simulink model "PONG"  (R2018b)
settings: Solver=VariableStepAuto  StartTime=0.0  StopTime=10  RelTol=1e-3
libraries: simulink_extras x28
(part 3 of 3)

== system PONG/Paddle DEMUXER1/1PaddleDEMUXER2 ==
  PA : Inport
  PB : Inport  Port=2
  PC : Inport  Port=3
  Logical Operator{,1..7} (8 alike) : Logic  Inputs=3  IconShape=distinctive  AllPortsSameDT=off  OutDataTypeStr=boolean
  NOT : Logic  Operator=NOT  IconShape=distinctive  AllPortsSameDT=off  OutDataTypeStr=boolean
  NOT1 : Logic  Operator=NOT  IconShape=distinctive  AllPortsSameDT=off  OutDataTypeStr=boolean
  NOT2 : Logic  Operator=NOT  IconShape=distinctive  AllPortsSameDT=off  OutDataTypeStr=boolean
  Out1 : Outport
  Out2 : Outport  Port=2
  Out3 : Outport  Port=3
  Out4 : Outport  Port=4
  Out5 : Outport  Port=5
  Out6 : Outport  Port=6
  Out7 : Outport  Port=7
  Out8 : Outport  Port=8
  wires:
  PB/1 -> NOT1/1, Logical Operator3/2, Logical Operator7/2, Logical Operator6/2, Logical Operator2/2
  PC/1 -> NOT/1, Logical Operator1/3, Logical Operator3/3, Logical Operator5/3, Logical Operator7/1
  NOT2/1 -> Logical Operator1/1, Logical Operator2/1, Logical Operator3/1, Logical Operator/1
  NOT1/1 -> Logical Operator/2, Logical Operator1/2, Logical Operator4/2, Logical Operator5/2
  NOT/1 -> Logical Operator4/3, Logical Operator6/3, Logical Operator2/3, Logical Operator/3
  PA/1 -> NOT2/1, Logical Operator4/1, Logical Operator5/1, Logical Operator7/3, Logical Operator6/1
  Logical Operator4/1 -> Out5/1
  Logical Operator5/1 -> Out6/1
  Logical Operator6/1 -> Out7/1
  Logical Operator7/1 -> Out8/1
  Logical Operator2/1 -> Out3/1
  Logical Operator3/1 -> Out4/1
  Logical Operator1/1 -> Out2/1
  Logical Operator/1 -> Out1/1

== system PONG/Paddle0/Atomic Subsystem ==
  Ctrl : Inport
  CLK : Inport  Port=2
  Constant : Constant  OutDataTypeStr=boolean
  J-K Flip-Flop : simulink_extras/Flip Flops/J-K Flip-Flop  initial_condition=0
      settings: SourceProductName=Simulink
  J-K Flip-Flop1 : simulink_extras/Flip Flops/J-K Flip-Flop  initial_condition=0
      settings: SourceProductName=Simulink
  J-K Flip-Flop2 : simulink_extras/Flip Flops/J-K Flip-Flop  initial_condition=0
      settings: SourceProductName=Simulink
  Logical Operator : Logic  Operator=XOR  IconShape=distinctive  AllPortsSameDT=off  OutDataTypeStr=boolean
  Logical Operator1 : Logic  Operator=XOR  IconShape=distinctive  AllPortsSameDT=off  OutDataTypeStr=boolean
  Scope : Scope  NumInputPorts=3
  PA0 : Outport
  PB0 : Outport  Port=2
  PC0 : Outport  Port=3
  wires:
  CLK/1 -> J-K Flip-Flop/2
  J-K Flip-Flop/1 -> Logical Operator/1, Scope/1, PC0/1
  J-K Flip-Flop2/1 -> Scope/3, PA0/1
  J-K Flip-Flop1/1 -> Logical Operator1/1, Scope/2, PB0/1
  Ctrl/1 -> Logical Operator1/2, Logical Operator/2
  Logical Operator/1 -> J-K Flip-Flop1/2
  Logical Operator1/1 -> J-K Flip-Flop2/2
  Constant/1 -> J-K Flip-Flop2/3, J-K Flip-Flop2/1, J-K Flip-Flop1/3, J-K Flip-Flop1/1, J-K Flip-Flop/3, J-K Flip-Flop/1

== system PONG/Paddle0/Atomic Subsystem1 ==
  PA0 : Inport
  PB0 : Inport  Port=2
  PC0 : Inport  Port=3
  Logical Operator1 : Logic  Operator=XOR  IconShape=distinctive  AllPortsSameDT=off  OutDataTypeStr=boolean
  Logical Operator2 : Logic  Operator=NOT  IconShape=distinctive  AllPortsSameDT=off  OutDataTypeStr=boolean
  Logical Operator3 : Logic  Operator=XOR  IconShape=distinctive  AllPortsSameDT=off  OutDataTypeStr=boolean
  Logical Operator4 : Logic  IconShape=distinctive  AllPortsSameDT=off  OutDataTypeStr=boolean
  Scope : Scope  NumInputPorts=3
  PA1 : Outport
  PB1 : Outport  Port=2
  PC1 : Outport  Port=3
  wires:
  Logical Operator2/1 -> Scope/3, PC1/1
  PB0/1 -> Logical Operator4/1, Logical Operator1/1
  PA0/1 -> Logical Operator3/1
  Logical Operator3/1 -> Scope/1, PA1/1
  Logical Operator1/1 -> Scope/2, PB1/1
  Logical Operator4/1 -> Logical Operator3/2
  PC0/1 -> Logical Operator4/2, Logical Operator1/2, Logical Operator2/1

== system PONG/Paddle0/Atomic Subsystem2 ==
  PA0 : Inport
  PB0 : Inport  Port=2
  PC0 : Inport  Port=3
  Logical Operator1 : Logic  Operator=NXOR  IconShape=distinctive  AllPortsSameDT=off  OutDataTypeStr=boolean
  Logical Operator2 : Logic  Operator=NOT  IconShape=distinctive  AllPortsSameDT=off  OutDataTypeStr=boolean
  Logical Operator3 : Logic  Operator=NXOR  IconShape=distinctive  AllPortsSameDT=off  OutDataTypeStr=boolean
  Logical Operator4 : Logic  Operator=OR  IconShape=distinctive  AllPortsSameDT=off  OutDataTypeStr=boolean
  Scope : Scope  NumInputPorts=3
  PA1 : Outport
  PB1 : Outport  Port=2
  PC1 : Outport  Port=3
  wires:
  PC0/1 -> Logical Operator2/1, Logical Operator1/2, Logical Operator4/2
  Logical Operator4/1 -> Logical Operator3/2
  Logical Operator1/1 -> PB1/1, Scope/2
  Logical Operator3/1 -> PA1/1, Scope/1
  PA0/1 -> Logical Operator3/1
  PB0/1 -> Logical Operator1/1, Logical Operator4/1
  Logical Operator2/1 -> PC1/1, Scope/3

== system PONG/Paddle0/Atomic Subsystem3 ==
  CLK : Inport
  Ctrl : Inport  Port=2
  Constant : Constant  OutDataTypeStr=boolean
  J-K Flip-Flop : simulink_extras/Flip Flops/J-K Flip-Flop  initial_condition=0
      settings: SourceProductName=Simulink
  J-K Flip-Flop1 : simulink_extras/Flip Flops/J-K Flip-Flop  initial_condition=0
      settings: SourceProductName=Simulink
  J-K Flip-Flop2 : simulink_extras/Flip Flops/J-K Flip-Flop  initial_condition=1
      settings: SourceProductName=Simulink
  Logical Operator12 : Logic  Operator=OR  IconShape=distinctive  AllPortsSameDT=off  OutDataTypeStr=boolean
  Logical Operator13 : Logic  Operator=OR  IconShape=distinctive  AllPortsSameDT=off  OutDataTypeStr=boolean
  Logical Operator{8..9,14..15} (4 alike) : Logic  IconShape=distinctive  AllPortsSameDT=off  OutDataTypeStr=boolean
  NOT1 : Logic  Operator=NOT  IconShape=distinctive  AllPortsSameDT=off  OutDataTypeStr=boolean
  Scope : Scope  NumInputPorts=3
  PA0 : Outport
  PB0 : Outport  Port=2
  PC0 : Outport  Port=3
  wires:
  J-K Flip-Flop1/2 -> Logical Operator15/1
  Logical Operator12/1 -> J-K Flip-Flop1/3, J-K Flip-Flop1/1
  Logical Operator8/1 -> Logical Operator12/1, Logical Operator14/1
  J-K Flip-Flop2/1 -> PA0/1, Scope/3
  J-K Flip-Flop1/1 -> Scope/2, PB0/1, Logical Operator14/2
  NOT1/1 -> Logical Operator9/2
  Logical Operator13/1 -> J-K Flip-Flop2/1, J-K Flip-Flop2/3
  Logical Operator9/1 -> Logical Operator15/2, Logical Operator12/2
  Logical Operator14/1 -> Logical Operator13/1
  Constant/1 -> J-K Flip-Flop/1, J-K Flip-Flop/3
  CLK/1 -> J-K Flip-Flop2/2, J-K Flip-Flop1/2, J-K Flip-Flop/2
  Ctrl/1 -> Logical Operator8/1, NOT1/1
  J-K Flip-Flop/1 -> Scope/1, PC0/1, Logical Operator8/2
  Logical Operator15/1 -> Logical Operator13/2
  J-K Flip-Flop/2 -> Logical Operator9/1

== system PONG/Paddle1/Atomic Subsystem1 ==
  PA0 : Inport
  PB0 : Inport  Port=2
  PC0 : Inport  Port=3
  Logical Operator1 : Logic  Operator=XOR  IconShape=distinctive  AllPortsSameDT=off  OutDataTypeStr=boolean
  Logical Operator2 : Logic  Operator=NOT  IconShape=distinctive  AllPortsSameDT=off  OutDataTypeStr=boolean
  Logical Operator3 : Logic  Operator=XOR  IconShape=distinctive  AllPortsSameDT=off  OutDataTypeStr=boolean
  Logical Operator4 : Logic  IconShape=distinctive  AllPortsSameDT=off  OutDataTypeStr=boolean
  Scope : Scope  NumInputPorts=3
  PA1 : Outport
  PB1 : Outport  Port=2
  PC1 : Outport  Port=3
  wires:
  PC0/1 -> Logical Operator2/1, Logical Operator1/2, Logical Operator4/2
  Logical Operator4/1 -> Logical Operator3/2
  Logical Operator1/1 -> PB1/1, Scope/2
  Logical Operator3/1 -> PA1/1, Scope/1
  PA0/1 -> Logical Operator3/1
  PB0/1 -> Logical Operator1/1, Logical Operator4/1
  Logical Operator2/1 -> PC1/1, Scope/3

== system PONG/Paddle1/Atomic Subsystem2 ==
  PA0 : Inport
  PB0 : Inport  Port=2
  PC0 : Inport  Port=3
  Logical Operator1 : Logic  Operator=NXOR  IconShape=distinctive  AllPortsSameDT=off  OutDataTypeStr=boolean
  Logical Operator2 : Logic  Operator=NOT  IconShape=distinctive  AllPortsSameDT=off  OutDataTypeStr=boolean
  Logical Operator3 : Logic  Operator=NXOR  IconShape=distinctive  AllPortsSameDT=off  OutDataTypeStr=boolean
  Logical Operator4 : Logic  Operator=OR  IconShape=distinctive  AllPortsSameDT=off  OutDataTypeStr=boolean
  Scope : Scope  NumInputPorts=3
  PA1 : Outport
  PB1 : Outport  Port=2
  PC1 : Outport  Port=3
  wires:
  Logical Operator2/1 -> Scope/3, PC1/1
  PB0/1 -> Logical Operator4/1, Logical Operator1/1
  PA0/1 -> Logical Operator3/1
  Logical Operator3/1 -> Scope/1, PA1/1
  Logical Operator1/1 -> Scope/2, PB1/1
  Logical Operator4/1 -> Logical Operator3/2
  PC0/1 -> Logical Operator4/2, Logical Operator1/2, Logical Operator2/1

== system PONG/Paddle1/Atomic Subsystem3 ==
  CLK : Inport
  Ctrl : Inport  Port=2
  Constant : Constant  OutDataTypeStr=boolean
  J-K Flip-Flop : simulink_extras/Flip Flops/J-K Flip-Flop  initial_condition=1
      settings: SourceProductName=Simulink
  J-K Flip-Flop1 : simulink_extras/Flip Flops/J-K Flip-Flop  initial_condition=1
      settings: SourceProductName=Simulink
  J-K Flip-Flop2 : simulink_extras/Flip Flops/J-K Flip-Flop  initial_condition=0
      settings: SourceProductName=Simulink
  Logical Operator12 : Logic  Operator=OR  IconShape=distinctive  AllPortsSameDT=off  OutDataTypeStr=boolean
  Logical Operator13 : Logic  Operator=OR  IconShape=distinctive  AllPortsSameDT=off  OutDataTypeStr=boolean
  Logical Operator{8..9,14..15} (4 alike) : Logic  IconShape=distinctive  AllPortsSameDT=off  OutDataTypeStr=boolean
  NOT1 : Logic  Operator=NOT  IconShape=distinctive  AllPortsSameDT=off  OutDataTypeStr=boolean
  Scope : Scope  NumInputPorts=3
  PA0 : Outport
  PB0 : Outport  Port=2
  PC0 : Outport  Port=3
  wires:
  J-K Flip-Flop/2 -> Logical Operator9/1
  Logical Operator15/1 -> Logical Operator13/2
  J-K Flip-Flop/1 -> Logical Operator8/2, PC0/1, Scope/1
  Ctrl/1 -> NOT1/1, Logical Operator8/1
  CLK/1 -> J-K Flip-Flop/2, J-K Flip-Flop1/2, J-K Flip-Flop2/2
  Constant/1 -> J-K Flip-Flop/3, J-K Flip-Flop/1
  Logical Operator14/1 -> Logical Operator13/1
  Logical Operator9/1 -> Logical Operator15/2, Logical Operator12/2
  Logical Operator13/1 -> J-K Flip-Flop2/3, J-K Flip-Flop2/1
  NOT1/1 -> Logical Operator9/2
  J-K Flip-Flop1/1 -> Logical Operator14/2, PB0/1, Scope/2
  J-K Flip-Flop2/1 -> Scope/3, PA0/1
  Logical Operator8/1 -> Logical Operator14/1, Logical Operator12/1
  Logical Operator12/1 -> J-K Flip-Flop1/1, J-K Flip-Flop1/3
  J-K Flip-Flop1/2 -> Logical Operator15/1

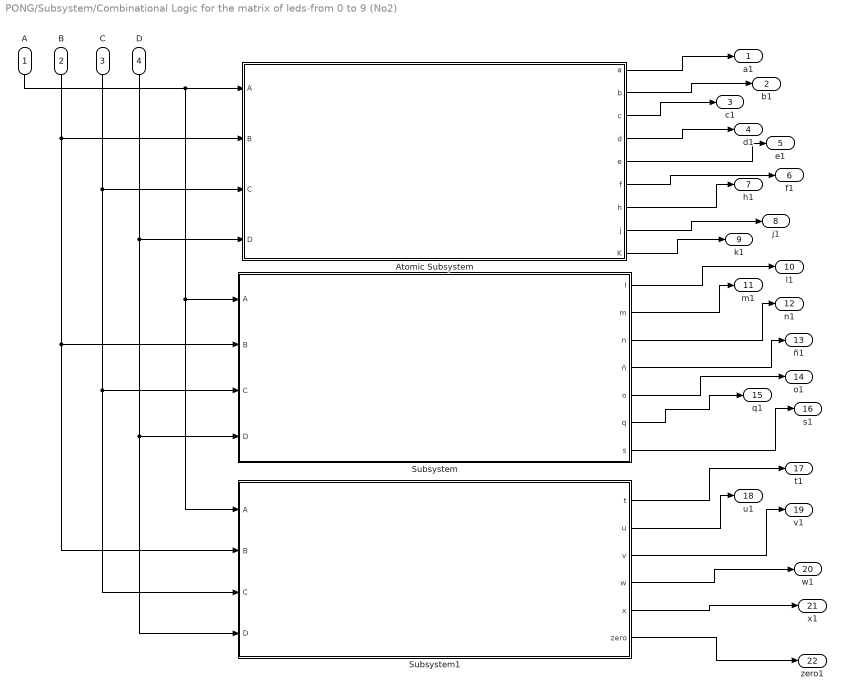
== system PONG/Subsystem/Combinational Logic for the matrix of leds-from 0 to 9 (No2) ==
  A : Inport
  B : Inport  Port=2
  C : Inport  Port=3
  D : Inport  Port=4
  Atomic Subsystem : Subsystem  TreatAsAtomicUnit=on
  Subsystem : Subsystem
  Subsystem1 : Subsystem
  a1 : Outport
  b1 : Outport  Port=2
  c1 : Outport  Port=3
  d1 : Outport  Port=4
  e1 : Outport  Port=5
  f1 : Outport  Port=6
  h1 : Outport  Port=7
  j1 : Outport  Port=8
  k1 : Outport  Port=9
  l1 : Outport  Port=10
  m1 : Outport  Port=11
  n1 : Outport  Port=12
  ñ1 : Outport  Port=13
  o1 : Outport  Port=14
  q1 : Outport  Port=15
  s1 : Outport  Port=16
  t1 : Outport  Port=17
  u1 : Outport  Port=18
  v1 : Outport  Port=19
  w1 : Outport  Port=20
  x1 : Outport  Port=21
  zero1 : Outport  Port=22
  wires:
  Atomic Subsystem/1(a) -> a1/1
  Atomic Subsystem/2(b) -> b1/1
  Atomic Subsystem/3(c) -> c1/1
  Atomic Subsystem/4(d) -> d1/1
  Atomic Subsystem/5(e) -> e1/1
  Atomic Subsystem/6(f) -> f1/1
  Atomic Subsystem/7(h) -> h1/1
  Atomic Subsystem/8(j) -> j1/1
  Atomic Subsystem/9(K) -> k1/1
  Subsystem/1(l) -> l1/1
  Subsystem/2(m) -> m1/1
  Subsystem/3(n) -> n1/1
  Subsystem/4(ñ) -> ñ1/1
  Subsystem/5(o) -> o1/1
  Subsystem/6(q) -> q1/1
  Subsystem/7(s) -> s1/1
  Subsystem1/1(t) -> t1/1
  Subsystem1/2(u) -> u1/1
  Subsystem1/3(v) -> v1/1
  Subsystem1/4(w) -> w1/1
  Subsystem1/5(x) -> x1/1
  A/1 -> Subsystem1/1(A), Subsystem/1(A), Atomic Subsystem/1(A)
  B/1 -> Subsystem1/2(B), Subsystem/2(B), Atomic Subsystem/2(B)
  C/1 -> Subsystem1/3(C), Subsystem/3(C), Atomic Subsystem/3(C)
  D/1 -> Subsystem1/4(D), Subsystem/4(D), Atomic Subsystem/4(D)
  Subsystem1/6(zero) -> zero1/1

== system PONG/Subsystem/Counter from 0 to 9 ==
  EN : Inport
  CLK : Inport  Port=2
  " B JK FLIP FLOP" : simulink_extras/Flip Flops/J-K Flip-Flop  initial_condition=0
      settings: SourceProductName=Simulink
  A JK FLIP FLOP : simulink_extras/Flip Flops/J-K Flip-Flop  initial_condition=0
      settings: SourceProductName=Simulink
  C Jk flip flop : simulink_extras/Flip Flops/J-K Flip-Flop  initial_condition=0
      settings: SourceProductName=Simulink
  D jk flip-flop : simulink_extras/Flip Flops/J-K Flip-Flop  initial_condition=0
      settings: SourceProductName=Simulink
  Display3 : Display
      settings: Format=binary (Stored Integer)
  Logical Operator : Logic  IconShape=distinctive  AllPortsSameDT=off  OutDataTypeStr=boolean
  Logical Operator1 : Logic  IconShape=distinctive  AllPortsSameDT=off  OutDataTypeStr=boolean
  Logical Operator2 : Logic  Inputs=3  IconShape=distinctive  AllPortsSameDT=off  OutDataTypeStr=boolean
  Mux : Mux
  A : Outport
  B : Outport  Port=2
  C : Outport  Port=3
  D : Outport  Port=4
  wires:
  C Jk flip flop/1 -> Logical Operator2/2, Logical Operator1/2, C/1, Mux/3
  Mux/1 -> Display3/1
  Logical Operator2/1 -> A JK FLIP FLOP/1
  A JK FLIP FLOP/1 -> A/1, Mux/1
  Logical Operator1/1 -> " B JK FLIP FLOP"/3, " B JK FLIP FLOP"/1
  Logical Operator/1 -> C Jk flip flop/1
  " B JK FLIP FLOP"/1 -> Logical Operator2/3, B/1, Mux/2
  CLK/1 -> A JK FLIP FLOP/2, " B JK FLIP FLOP"/2, C Jk flip flop/2, D jk flip-flop/2
  D jk flip-flop/1 -> Logical Operator2/1, A JK FLIP FLOP/3, Logical Operator1/1, Logical Operator/1, D/1, Mux/4, C Jk flip flop/3
  EN/1 -> D jk flip-flop/3, D jk flip-flop/1
  A JK FLIP FLOP/2 -> Logical Operator/2

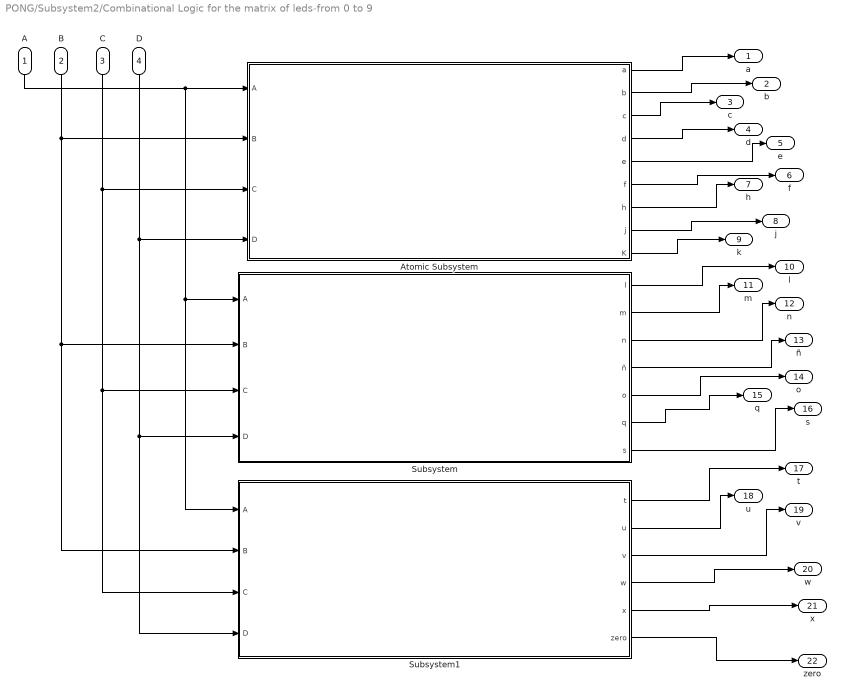
== system PONG/Subsystem2/Combinational Logic for the matrix of leds-from 0 to 9 ==
  A : Inport
  B : Inport  Port=2
  C : Inport  Port=3
  D : Inport  Port=4
  Atomic Subsystem : Subsystem  TreatAsAtomicUnit=on
  Subsystem : Subsystem
  Subsystem1 : Subsystem
  a : Outport
  b : Outport  Port=2
  c : Outport  Port=3
  d : Outport  Port=4
  e : Outport  Port=5
  f : Outport  Port=6
  h : Outport  Port=7
  j : Outport  Port=8
  k : Outport  Port=9
  l : Outport  Port=10
  m : Outport  Port=11
  n : Outport  Port=12
  ñ : Outport  Port=13
  o : Outport  Port=14
  q : Outport  Port=15
  s : Outport  Port=16
  t : Outport  Port=17
  u : Outport  Port=18
  v : Outport  Port=19
  w : Outport  Port=20
  x : Outport  Port=21
  zero : Outport  Port=22
  wires:
  Atomic Subsystem/1(a) -> a/1
  Atomic Subsystem/2(b) -> b/1
  Atomic Subsystem/3(c) -> c/1
  Atomic Subsystem/4(d) -> d/1
  Atomic Subsystem/5(e) -> e/1
  Atomic Subsystem/6(f) -> f/1
  Atomic Subsystem/7(h) -> h/1
  Atomic Subsystem/8(j) -> j/1
  Atomic Subsystem/9(K) -> k/1
  Subsystem/1(l) -> l/1
  Subsystem/2(m) -> m/1
  Subsystem/3(n) -> n/1
  Subsystem/4(ñ) -> ñ/1
  Subsystem/5(o) -> o/1
  Subsystem/6(q) -> q/1
  Subsystem/7(s) -> s/1
  Subsystem1/1(t) -> t/1
  Subsystem1/2(u) -> u/1
  Subsystem1/3(v) -> v/1
  Subsystem1/4(w) -> w/1
  Subsystem1/5(x) -> x/1
  A/1 -> Subsystem1/1(A), Subsystem/1(A), Atomic Subsystem/1(A)
  B/1 -> Subsystem1/2(B), Subsystem/2(B), Atomic Subsystem/2(B)
  C/1 -> Subsystem1/3(C), Subsystem/3(C), Atomic Subsystem/3(C)
  D/1 -> Subsystem1/4(D), Subsystem/4(D), Atomic Subsystem/4(D)
  Subsystem1/6(zero) -> zero/1

== system PONG/Subsystem2/Counter from 0 to 9 ==
  EN : Inport
  CLK : Inport  Port=2
  " B JK FLIP FLOP" : simulink_extras/Flip Flops/J-K Flip-Flop  initial_condition=0
      settings: SourceProductName=Simulink
  A JK FLIP FLOP : simulink_extras/Flip Flops/J-K Flip-Flop  initial_condition=0
      settings: SourceProductName=Simulink
  C Jk flip flop : simulink_extras/Flip Flops/J-K Flip-Flop  initial_condition=0
      settings: SourceProductName=Simulink
  D jk flip-flop : simulink_extras/Flip Flops/J-K Flip-Flop  initial_condition=0
      settings: SourceProductName=Simulink
  Display3 : Display
      settings: Format=binary (Stored Integer)
  Logical Operator : Logic  IconShape=distinctive  AllPortsSameDT=off  OutDataTypeStr=boolean
  Logical Operator1 : Logic  IconShape=distinctive  AllPortsSameDT=off  OutDataTypeStr=boolean
  Logical Operator2 : Logic  Inputs=3  IconShape=distinctive  AllPortsSameDT=off  OutDataTypeStr=boolean
  Mux : Mux
  A : Outport
  B : Outport  Port=2
  C : Outport  Port=3
  D : Outport  Port=4
  wires:
  Mux/1 -> Display3/1
  D jk flip-flop/1 -> Logical Operator2/1, A JK FLIP FLOP/3, Logical Operator1/1, Logical Operator/1, D/1, Mux/4, C Jk flip flop/3
  C Jk flip flop/1 -> Logical Operator2/2, Logical Operator1/2, C/1, Mux/3
  EN/1 -> D jk flip-flop/3, D jk flip-flop/1
  A JK FLIP FLOP/1 -> A/1, Mux/1
  A JK FLIP FLOP/2 -> Logical Operator/2
  Logical Operator/1 -> C Jk flip flop/1
  Logical Operator1/1 -> " B JK FLIP FLOP"/3, " B JK FLIP FLOP"/1
  " B JK FLIP FLOP"/1 -> Logical Operator2/3, B/1, Mux/2
  Logical Operator2/1 -> A JK FLIP FLOP/1
  CLK/1 -> A JK FLIP FLOP/2, " B JK FLIP FLOP"/2, C Jk flip flop/2, D jk flip-flop/2

== system PONG/Next State /MOVE_XBall_CONTROLLED ( EN=0 >Right ;  EN=1 > left ) 3/Reset_Control1 ==
  EN_reset : Inport
  "JK " : Inport  Port=2
  A' : Inport  Port=3
  Logical Operator{,1..3} (4 alike) : Logic  IconShape=distinctive  AllPortsSameDT=off  OutDataTypeStr=boolean
  Logical Operator4 : Logic  Operator=OR  IconShape=distinctive  AllPortsSameDT=off  OutDataTypeStr=boolean
  Logical Operator5 : Logic  Operator=OR  IconShape=distinctive  AllPortsSameDT=off  OutDataTypeStr=boolean
  Logical Operator6 : Logic  Operator=NOT  IconShape=distinctive  AllPortsSameDT=off  OutDataTypeStr=boolean
  Logical Operator7 : Logic  Operator=NOT  IconShape=distinctive  AllPortsSameDT=off  OutDataTypeStr=boolean
  Logical Operator8 : Logic  Operator=NOT  IconShape=distinctive  AllPortsSameDT=off  OutDataTypeStr=boolean
  J : Outport
  K : Outport  Port=2
  wires:
  "JK "/1 -> Logical Operator1/2, Logical Operator/2
  Logical Operator8/1 -> Logical Operator3/2
  Logical Operator7/1 -> Logical Operator1/1
  Logical Operator6/1 -> Logical Operator/1
  A'/1 -> Logical Operator8/1, Logical Operator2/2
  Logical Operator2/1 -> Logical Operator4/2
  Logical Operator1/1 -> Logical Operator5/1
  Logical Operator/1 -> Logical Operator4/1
  Logical Operator3/1 -> Logical Operator5/2
  Logical Operator5/1 -> K/1
  Logical Operator4/1 -> J/1
  EN_reset/1 -> Logical Operator6/1, Logical Operator7/1, Logical Operator2/1, Logical Operator3/1

== system PONG/Next State /MOVE_XBall_CONTROLLED ( EN=0 >Right ;  EN=1 > left ) 3/Reset_Control2 ==
  EN_reset : Inport
  "JK " : Inport  Port=2
  Logical Operator : Logic  IconShape=distinctive  AllPortsSameDT=off  OutDataTypeStr=boolean
  Logical Operator1 : Logic  IconShape=distinctive  AllPortsSameDT=off  OutDataTypeStr=boolean
  Logical Operator6 : Logic  Operator=NOT  IconShape=distinctive  AllPortsSameDT=off  OutDataTypeStr=boolean
  Logical Operator7 : Logic  Operator=NOT  IconShape=distinctive  AllPortsSameDT=off  OutDataTypeStr=boolean
  J : Outport
  K : Outport  Port=2
  wires:
  "JK "/1 -> Logical Operator1/2, Logical Operator/2
  Logical Operator7/1 -> Logical Operator1/1
  Logical Operator6/1 -> Logical Operator/1
  Logical Operator1/1 -> K/1
  Logical Operator/1 -> J/1
  EN_reset/1 -> Logical Operator6/1, Logical Operator7/1

== system PONG/Next State /MOVE_XBall_CONTROLLED ( EN=0 >Right ;  EN=1 > left ) 3/Reset_Control3 ==
  EN_reset : Inport
  "JK " : Inport  Port=2
  A' : Inport  Port=3
  Logical Operator{,1..3} (4 alike) : Logic  IconShape=distinctive  AllPortsSameDT=off  OutDataTypeStr=boolean
  Logical Operator4 : Logic  Operator=OR  IconShape=distinctive  AllPortsSameDT=off  OutDataTypeStr=boolean
  Logical Operator5 : Logic  Operator=OR  IconShape=distinctive  AllPortsSameDT=off  OutDataTypeStr=boolean
  Logical Operator6 : Logic  Operator=NOT  IconShape=distinctive  AllPortsSameDT=off  OutDataTypeStr=boolean
  Logical Operator7 : Logic  Operator=NOT  IconShape=distinctive  AllPortsSameDT=off  OutDataTypeStr=boolean
  Logical Operator8 : Logic  Operator=NOT  IconShape=distinctive  AllPortsSameDT=off  OutDataTypeStr=boolean
  J : Outport
  K : Outport  Port=2
  wires:
  "JK "/1 -> Logical Operator1/2, Logical Operator/2
  Logical Operator8/1 -> Logical Operator3/2
  Logical Operator7/1 -> Logical Operator1/1
  Logical Operator6/1 -> Logical Operator/1
  A'/1 -> Logical Operator8/1, Logical Operator2/2
  Logical Operator2/1 -> Logical Operator4/2
  Logical Operator1/1 -> Logical Operator5/1
  Logical Operator/1 -> Logical Operator4/1
  Logical Operator3/1 -> Logical Operator5/2
  Logical Operator5/1 -> K/1
  Logical Operator4/1 -> J/1
  EN_reset/1 -> Logical Operator6/1, Logical Operator7/1, Logical Operator2/1, Logical Operator3/1

== system PONG/Next State /MOVE_XBall_CONTROLLED ( EN=0 >Right ;  EN=1 > left ) 3/Reset_Control4 ==
  EN_reset : Inport
  "JK " : Inport  Port=2
  A' : Inport  Port=3
  Logical Operator{,1..3} (4 alike) : Logic  IconShape=distinctive  AllPortsSameDT=off  OutDataTypeStr=boolean
  Logical Operator4 : Logic  Operator=OR  IconShape=distinctive  AllPortsSameDT=off  OutDataTypeStr=boolean
  Logical Operator5 : Logic  Operator=OR  IconShape=distinctive  AllPortsSameDT=off  OutDataTypeStr=boolean
  Logical Operator6 : Logic  Operator=NOT  IconShape=distinctive  AllPortsSameDT=off  OutDataTypeStr=boolean
  Logical Operator7 : Logic  Operator=NOT  IconShape=distinctive  AllPortsSameDT=off  OutDataTypeStr=boolean
  Logical Operator8 : Logic  Operator=NOT  IconShape=distinctive  AllPortsSameDT=off  OutDataTypeStr=boolean
  J : Outport
  K : Outport  Port=2
  wires:
  "JK "/1 -> Logical Operator1/2, Logical Operator/2
  Logical Operator8/1 -> Logical Operator3/2
  Logical Operator7/1 -> Logical Operator1/1
  Logical Operator6/1 -> Logical Operator/1
  A'/1 -> Logical Operator8/1, Logical Operator2/2
  Logical Operator2/1 -> Logical Operator4/2
  Logical Operator1/1 -> Logical Operator5/1
  Logical Operator/1 -> Logical Operator4/1
  Logical Operator3/1 -> Logical Operator5/2
  Logical Operator5/1 -> K/1
  Logical Operator4/1 -> J/1
  EN_reset/1 -> Logical Operator6/1, Logical Operator7/1, Logical Operator2/1, Logical Operator3/1

== system PONG/Next State /MOVE_YBall_CONTROLLED ( EN=0 >Up ;  EN=1 > Down ) 3/Reset_Control ==
  EN_reset : Inport
  "JK " : Inport  Port=2
  E' : Inport  Port=3
  Logical Operator{,1..3} (4 alike) : Logic  IconShape=distinctive  AllPortsSameDT=off  OutDataTypeStr=boolean
  Logical Operator4 : Logic  Operator=OR  IconShape=distinctive  AllPortsSameDT=off  OutDataTypeStr=boolean
  Logical Operator5 : Logic  Operator=OR  IconShape=distinctive  AllPortsSameDT=off  OutDataTypeStr=boolean
  Logical Operator6 : Logic  Operator=NOT  IconShape=distinctive  AllPortsSameDT=off  OutDataTypeStr=boolean
  Logical Operator7 : Logic  Operator=NOT  IconShape=distinctive  AllPortsSameDT=off  OutDataTypeStr=boolean
  Logical Operator8 : Logic  Operator=NOT  IconShape=distinctive  AllPortsSameDT=off  OutDataTypeStr=boolean
  J : Outport
  K : Outport  Port=2
  wires:
  EN_reset/1 -> Logical Operator3/1, Logical Operator2/1, Logical Operator7/1, Logical Operator6/1
  Logical Operator4/1 -> J/1
  Logical Operator5/1 -> K/1
  Logical Operator3/1 -> Logical Operator5/2
  Logical Operator/1 -> Logical Operator4/1
  Logical Operator1/1 -> Logical Operator5/1
  Logical Operator2/1 -> Logical Operator4/2
  E'/1 -> Logical Operator2/2, Logical Operator8/1
  Logical Operator6/1 -> Logical Operator/1
  Logical Operator7/1 -> Logical Operator1/1
  Logical Operator8/1 -> Logical Operator3/2
  "JK "/1 -> Logical Operator/2, Logical Operator1/2

== system PONG/Next State /MOVE_YBall_CONTROLLED ( EN=0 >Up ;  EN=1 > Down ) 3/Reset_Control1 ==
  EN_reset : Inport
  "JK " : Inport  Port=2
  E' : Inport  Port=3
  Logical Operator{,1..3} (4 alike) : Logic  IconShape=distinctive  AllPortsSameDT=off  OutDataTypeStr=boolean
  Logical Operator4 : Logic  Operator=OR  IconShape=distinctive  AllPortsSameDT=off  OutDataTypeStr=boolean
  Logical Operator5 : Logic  Operator=OR  IconShape=distinctive  AllPortsSameDT=off  OutDataTypeStr=boolean
  Logical Operator6 : Logic  Operator=NOT  IconShape=distinctive  AllPortsSameDT=off  OutDataTypeStr=boolean
  Logical Operator7 : Logic  Operator=NOT  IconShape=distinctive  AllPortsSameDT=off  OutDataTypeStr=boolean
  Logical Operator8 : Logic  Operator=NOT  IconShape=distinctive  AllPortsSameDT=off  OutDataTypeStr=boolean
  J : Outport
  K : Outport  Port=2
  wires:
  "JK "/1 -> Logical Operator1/2, Logical Operator/2
  Logical Operator8/1 -> Logical Operator3/2
  Logical Operator7/1 -> Logical Operator1/1
  Logical Operator6/1 -> Logical Operator/1
  E'/1 -> Logical Operator8/1, Logical Operator2/2
  Logical Operator2/1 -> Logical Operator4/2
  Logical Operator1/1 -> Logical Operator5/1
  Logical Operator/1 -> Logical Operator4/1
  Logical Operator3/1 -> Logical Operator5/2
  Logical Operator5/1 -> K/1
  Logical Operator4/1 -> J/1
  EN_reset/1 -> Logical Operator6/1, Logical Operator7/1, Logical Operator2/1, Logical Operator3/1

== system PONG/Next State /MOVE_YBall_CONTROLLED ( EN=0 >Up ;  EN=1 > Down ) 3/Reset_Control2 ==
  EN_reset : Inport
  "JK " : Inport  Port=2
  Logical Operator : Logic  IconShape=distinctive  AllPortsSameDT=off  OutDataTypeStr=boolean
  Logical Operator1 : Logic  IconShape=distinctive  AllPortsSameDT=off  OutDataTypeStr=boolean
  Logical Operator6 : Logic  Operator=NOT  IconShape=distinctive  AllPortsSameDT=off  OutDataTypeStr=boolean
  Logical Operator7 : Logic  Operator=NOT  IconShape=distinctive  AllPortsSameDT=off  OutDataTypeStr=boolean
  J : Outport
  K : Outport  Port=2
  wires:
  "JK "/1 -> Logical Operator1/2, Logical Operator/2
  Logical Operator7/1 -> Logical Operator1/1
  Logical Operator6/1 -> Logical Operator/1
  Logical Operator1/1 -> K/1
  Logical Operator/1 -> J/1
  EN_reset/1 -> Logical Operator6/1, Logical Operator7/1

== system PONG/Paddle Control/Paddle Control0/Paddle Control0 ==
  E : Inport
  F : Inport  Port=2
  G : Inport  Port=3
  PA : Inport  Port=4
  PB : Inport  Port=5
  PC : Inport  Port=6
  Logical Operator : Logic  Inputs=3  IconShape=distinctive  AllPortsSameDT=off  OutDataTypeStr=boolean
  XOR : Logic  Operator=NXOR  IconShape=distinctive  AllPortsSameDT=off  OutDataTypeStr=boolean
  XOR1 : Logic  Operator=NXOR  IconShape=distinctive  AllPortsSameDT=off  OutDataTypeStr=boolean
  XOR2 : Logic  Operator=NXOR  IconShape=distinctive  AllPortsSameDT=off  OutDataTypeStr=boolean
  Out1 : Outport
  wires:
  Logical Operator/1 -> Out1/1
  XOR2/1 -> Logical Operator/3
  XOR1/1 -> Logical Operator/2
  XOR/1 -> Logical Operator/1
  E/1 -> XOR/1
  PA/1 -> XOR/2
  G/1 -> XOR2/1
  PC/1 -> XOR2/2
  PB/1 -> XOR1/2
  F/1 -> XOR1/1

== system PONG/Paddle Control/Paddle Control0/Paddle Control1 ==
  E : Inport
  F : Inport  Port=2
  G : Inport  Port=3
  PA : Inport  Port=4
  PB : Inport  Port=5
  PC : Inport  Port=6
  Logical Operator : Logic  Inputs=3  IconShape=distinctive  AllPortsSameDT=off  OutDataTypeStr=boolean
  XOR : Logic  Operator=NXOR  IconShape=distinctive  AllPortsSameDT=off  OutDataTypeStr=boolean
  XOR1 : Logic  Operator=NXOR  IconShape=distinctive  AllPortsSameDT=off  OutDataTypeStr=boolean
  XOR2 : Logic  Operator=NXOR  IconShape=distinctive  AllPortsSameDT=off  OutDataTypeStr=boolean
  Out1 : Outport
  wires:
  F/1 -> XOR1/1
  PB/1 -> XOR1/2
  PC/1 -> XOR2/2
  G/1 -> XOR2/1
  PA/1 -> XOR/2
  E/1 -> XOR/1
  XOR/1 -> Logical Operator/1
  XOR1/1 -> Logical Operator/2
  XOR2/1 -> Logical Operator/3
  Logical Operator/1 -> Out1/1

== system PONG/Paddle Control/Paddle Control0/Paddle Control2 ==
  E : Inport
  F : Inport  Port=2
  G : Inport  Port=3
  PA : Inport  Port=4
  PB : Inport  Port=5
  PC : Inport  Port=6
  Logical Operator : Logic  Inputs=3  IconShape=distinctive  AllPortsSameDT=off  OutDataTypeStr=boolean
  XOR : Logic  Operator=NXOR  IconShape=distinctive  AllPortsSameDT=off  OutDataTypeStr=boolean
  XOR1 : Logic  Operator=NXOR  IconShape=distinctive  AllPortsSameDT=off  OutDataTypeStr=boolean
  XOR2 : Logic  Operator=NXOR  IconShape=distinctive  AllPortsSameDT=off  OutDataTypeStr=boolean
  Out1 : Outport
  wires:
  Logical Operator/1 -> Out1/1
  XOR2/1 -> Logical Operator/3
  XOR1/1 -> Logical Operator/2
  XOR/1 -> Logical Operator/1
  E/1 -> XOR/1
  PA/1 -> XOR/2
  G/1 -> XOR2/1
  PC/1 -> XOR2/2
  PB/1 -> XOR1/2
  F/1 -> XOR1/1

== system PONG/Paddle Control/Paddle Control1/Paddle Control0 ==
  E : Inport
  F : Inport  Port=2
  G : Inport  Port=3
  PA : Inport  Port=4
  PB : Inport  Port=5
  PC : Inport  Port=6
  Logical Operator : Logic  Inputs=3  IconShape=distinctive  AllPortsSameDT=off  OutDataTypeStr=boolean
  XOR : Logic  Operator=NXOR  IconShape=distinctive  AllPortsSameDT=off  OutDataTypeStr=boolean
  XOR1 : Logic  Operator=NXOR  IconShape=distinctive  AllPortsSameDT=off  OutDataTypeStr=boolean
  XOR2 : Logic  Operator=NXOR  IconShape=distinctive  AllPortsSameDT=off  OutDataTypeStr=boolean
  Out1 : Outport
  wires:
  F/1 -> XOR1/1
  PB/1 -> XOR1/2
  PC/1 -> XOR2/2
  G/1 -> XOR2/1
  PA/1 -> XOR/2
  E/1 -> XOR/1
  XOR/1 -> Logical Operator/1
  XOR1/1 -> Logical Operator/2
  XOR2/1 -> Logical Operator/3
  Logical Operator/1 -> Out1/1

== system PONG/Paddle Control/Paddle Control1/Paddle Control1 ==
  E : Inport
  F : Inport  Port=2
  G : Inport  Port=3
  PA : Inport  Port=4
  PB : Inport  Port=5
  PC : Inport  Port=6
  Logical Operator : Logic  Inputs=3  IconShape=distinctive  AllPortsSameDT=off  OutDataTypeStr=boolean
  XOR : Logic  Operator=NXOR  IconShape=distinctive  AllPortsSameDT=off  OutDataTypeStr=boolean
  XOR1 : Logic  Operator=NXOR  IconShape=distinctive  AllPortsSameDT=off  OutDataTypeStr=boolean
  XOR2 : Logic  Operator=NXOR  IconShape=distinctive  AllPortsSameDT=off  OutDataTypeStr=boolean
  Out1 : Outport
  wires:
  Logical Operator/1 -> Out1/1
  XOR2/1 -> Logical Operator/3
  XOR1/1 -> Logical Operator/2
  XOR/1 -> Logical Operator/1
  E/1 -> XOR/1
  PA/1 -> XOR/2
  G/1 -> XOR2/1
  PC/1 -> XOR2/2
  PB/1 -> XOR1/2
  F/1 -> XOR1/1

== system PONG/Paddle Control/Paddle Control1/Paddle Control2 ==
  E : Inport
  F : Inport  Port=2
  G : Inport  Port=3
  PA : Inport  Port=4
  PB : Inport  Port=5
  PC : Inport  Port=6
  Logical Operator : Logic  Inputs=3  IconShape=distinctive  AllPortsSameDT=off  OutDataTypeStr=boolean
  XOR : Logic  Operator=NXOR  IconShape=distinctive  AllPortsSameDT=off  OutDataTypeStr=boolean
  XOR1 : Logic  Operator=NXOR  IconShape=distinctive  AllPortsSameDT=off  OutDataTypeStr=boolean
  XOR2 : Logic  Operator=NXOR  IconShape=distinctive  AllPortsSameDT=off  OutDataTypeStr=boolean
  Out1 : Outport
  wires:
  F/1 -> XOR1/1
  PB/1 -> XOR1/2
  PC/1 -> XOR2/2
  G/1 -> XOR2/1
  PA/1 -> XOR/2
  E/1 -> XOR/1
  XOR/1 -> Logical Operator/1
  XOR1/1 -> Logical Operator/2
  XOR2/1 -> Logical Operator/3
  Logical Operator/1 -> Out1/1

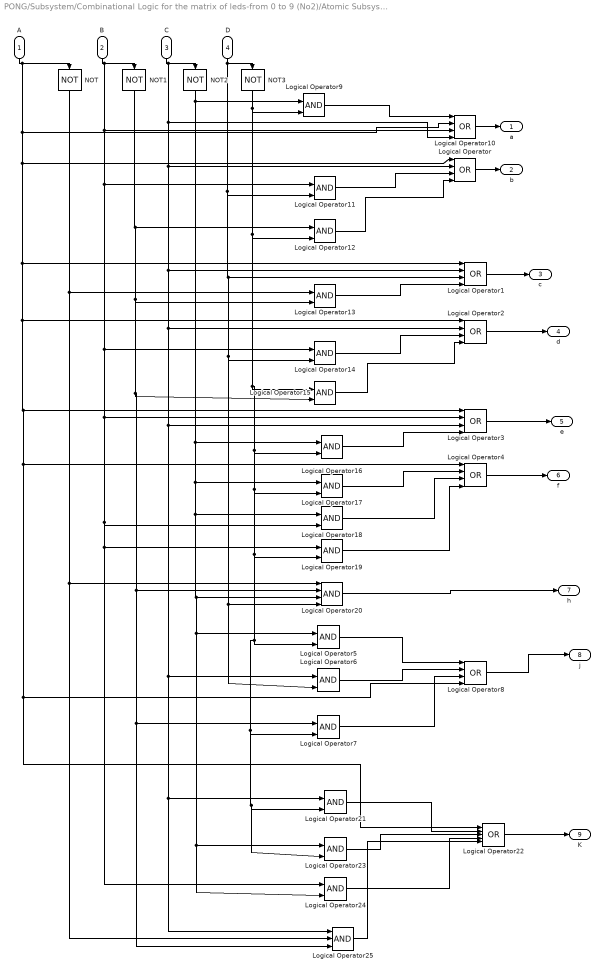
== system PONG/Subsystem/Combinational Logic for the matrix of leds-from 0 to 9 (No2)/Atomic Subsystem ==
  A : Inport
  B : Inport  Port=2
  C : Inport  Port=3
  D : Inport  Port=4
  Logical Operator{,1..4,8,10} (7 alike) : Logic  Operator=OR  Inputs=4  IconShape=distinctive  AllPortsSameDT=off  OutDataTypeStr=boolean
  Logical Operator{5..7,9,11..19,21,23..24} (16 alike) : Logic  IconShape=distinctive  AllPortsSameDT=off  OutDataTypeStr=boolean
  Logical Operator20 : Logic  Inputs=4  IconShape=distinctive  AllPortsSameDT=off  OutDataTypeStr=boolean
  Logical Operator22 : Logic  Operator=OR  Inputs=5  IconShape=distinctive  AllPortsSameDT=off  OutDataTypeStr=boolean
  Logical Operator25 : Logic  Inputs=3  IconShape=distinctive  AllPortsSameDT=off  OutDataTypeStr=boolean
  NOT{,1..3} (4 alike) : Logic  Operator=NOT  IconShape=distinctive  AllPortsSameDT=off  OutDataTypeStr=boolean
  a : Outport
  b : Outport  Port=2
  c : Outport  Port=3
  d : Outport  Port=4
  e : Outport  Port=5
  f : Outport  Port=6
  h : Outport  Port=7
  j : Outport  Port=8
  K : Outport  Port=9
  wires:
  Logical Operator8/1 -> j/1
  Logical Operator20/1 -> h/1
  Logical Operator12/1 -> Logical Operator/4
  A/1 -> Logical Operator8/4, Logical Operator22/1, Logical Operator4/1, Logical Operator3/1, Logical Operator2/1, Logical Operator1/1, Logical Operator/1, Logical Operator10/2, NOT/1
  Logical Operator3/1 -> e/1
  NOT1/1 -> Logical Operator25/3, Logical Operator7/1, Logical Operator20/2, Logical Operator15/2, Logical Operator13/2, Logical Operator12/1
  B/1 -> Logical Operator24/1, Logical Operator19/1, Logical Operator18/2, Logical Operator3/2, Logical Operator14/1, Logical Operator11/1, Logical Operator10/3, NOT1/1
  Logical Operator1/1 -> c/1
  Logical Operator4/1 -> f/1
  NOT2/1 -> Logical Operator24/2, Logical Operator23/1, Logical Operator5/1, Logical Operator20/3, Logical Operator18/1, Logical Operator17/1, Logical Operator16/1, Logical Operator9/1
  NOT3/1 -> Logical Operator19/2, Logical Operator23/2, Logical Operator21/2, Logical Operator7/2, Logical Operator5/2, Logical Operator17/2, Logical Operator16/2, Logical Operator15/1, Logical Operator12/2, Logical Operator9/2
  Logical Operator11/1 -> Logical Operator/3
  Logical Operator2/1 -> d/1
  D/1 -> Logical Operator6/2, Logical Operator20/4, Logical Operator14/2, Logical Operator1/3, Logical Operator11/2, NOT3/1
  Logical Operator9/1 -> Logical Operator10/1
  NOT/1 -> Logical Operator25/2, Logical Operator20/1, Logical Operator13/1
  Logical Operator13/1 -> Logical Operator1/4
  Logical Operator10/1 -> a/1
  Logical Operator/1 -> b/1
  Logical Operator14/1 -> Logical Operator2/3
  Logical Operator15/1 -> Logical Operator2/4
  Logical Operator16/1 -> Logical Operator3/4
  Logical Operator17/1 -> Logical Operator4/2
  Logical Operator18/1 -> Logical Operator4/3
  Logical Operator19/1 -> Logical Operator4/4
  Logical Operator5/1 -> Logical Operator8/1
  Logical Operator6/1 -> Logical Operator8/2
  Logical Operator7/1 -> Logical Operator8/3
  Logical Operator21/1 -> Logical Operator22/2
  Logical Operator23/1 -> Logical Operator22/3
  Logical Operator24/1 -> Logical Operator22/4
  Logical Operator22/1 -> K/1
  C/1 -> Logical Operator25/1, Logical Operator21/1, Logical Operator6/1, Logical Operator3/3, Logical Operator2/2, Logical Operator1/2, Logical Operator/2, Logical Operator10/4, NOT2/1
  Logical Operator25/1 -> Logical Operator22/5

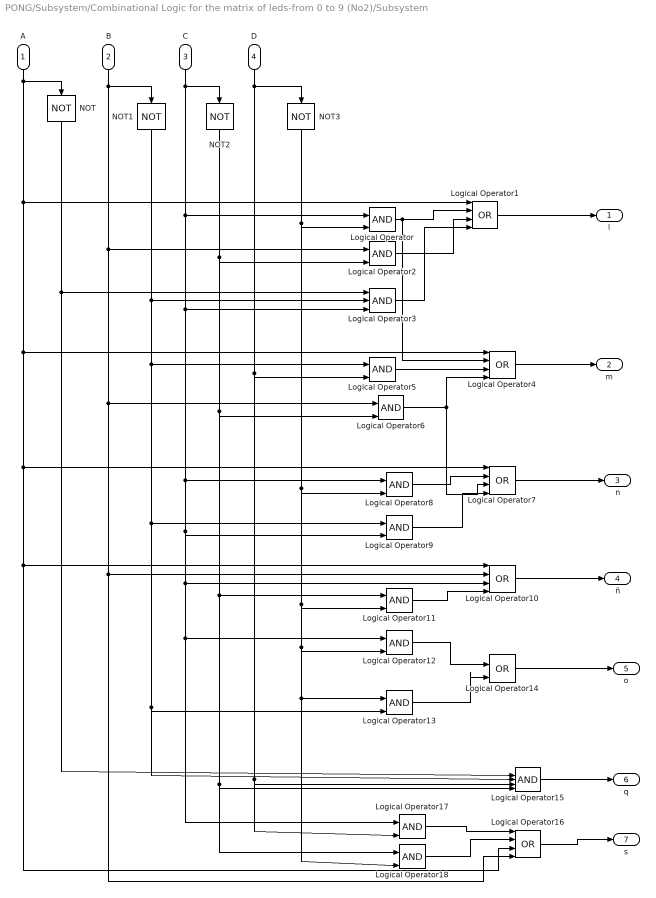
== system PONG/Subsystem/Combinational Logic for the matrix of leds-from 0 to 9 (No2)/Subsystem ==
  A : Inport
  B : Inport  Port=2
  C : Inport  Port=3
  D : Inport  Port=4
  Logical Operator{,2,5..6,8..9,11..13,17..18} (11 alike) : Logic  IconShape=distinctive  AllPortsSameDT=off  OutDataTypeStr=boolean
  Logical Operator{1,4,7,10,16} (5 alike) : Logic  Operator=OR  Inputs=4  IconShape=distinctive  AllPortsSameDT=off  OutDataTypeStr=boolean
  Logical Operator14 : Logic  Operator=OR  IconShape=distinctive  AllPortsSameDT=off  OutDataTypeStr=boolean
  Logical Operator15 : Logic  Inputs=4  IconShape=distinctive  AllPortsSameDT=off  OutDataTypeStr=boolean
  Logical Operator3 : Logic  Inputs=3  IconShape=distinctive  AllPortsSameDT=off  OutDataTypeStr=boolean
  NOT{,1..3} (4 alike) : Logic  Operator=NOT  IconShape=distinctive  AllPortsSameDT=off  OutDataTypeStr=boolean
  l : Outport
  m : Outport  Port=2
  n : Outport  Port=3
  ñ : Outport  Port=4
  o : Outport  Port=5
  q : Outport  Port=6
  s : Outport  Port=7
  wires:
  B/1 -> Logical Operator16/4, Logical Operator10/2, Logical Operator6/1, Logical Operator2/1, NOT1/1
  C/1 -> Logical Operator17/1, Logical Operator12/1, Logical Operator10/3, Logical Operator9/2, Logical Operator8/1, Logical Operator3/3, Logical Operator/1, NOT2/1
  D/1 -> Logical Operator17/2, Logical Operator15/3, Logical Operator5/2, NOT3/1
  NOT3/1 -> Logical Operator18/2, Logical Operator13/1, Logical Operator12/2, Logical Operator11/2, Logical Operator8/2, Logical Operator/2
  Logical Operator/1 -> Logical Operator4/2, Logical Operator1/2
  NOT2/1 -> Logical Operator18/1, Logical Operator15/4, Logical Operator11/1, Logical Operator6/2, Logical Operator2/2
  Logical Operator2/1 -> Logical Operator1/3
  NOT/1 -> Logical Operator15/1, Logical Operator3/1
  NOT1/1 -> Logical Operator15/2, Logical Operator13/2, Logical Operator9/1, Logical Operator5/1, Logical Operator3/2
  Logical Operator3/1 -> Logical Operator1/4
  A/1 -> Logical Operator16/3, Logical Operator10/1, Logical Operator7/1, Logical Operator4/1, Logical Operator1/1, NOT/1
  Logical Operator5/1 -> Logical Operator4/3
  Logical Operator6/1 -> Logical Operator7/3, Logical Operator4/4
  Logical Operator1/1 -> l/1
  Logical Operator4/1 -> m/1
  Logical Operator7/1 -> n/1
  Logical Operator8/1 -> Logical Operator7/2
  Logical Operator9/1 -> Logical Operator7/4
  Logical Operator11/1 -> Logical Operator10/4
  Logical Operator10/1 -> ñ/1
  Logical Operator12/1 -> Logical Operator14/1
  Logical Operator13/1 -> Logical Operator14/2
  Logical Operator14/1 -> o/1
  Logical Operator15/1 -> q/1
  Logical Operator17/1 -> Logical Operator16/1
  Logical Operator18/1 -> Logical Operator16/2
  Logical Operator16/1 -> s/1

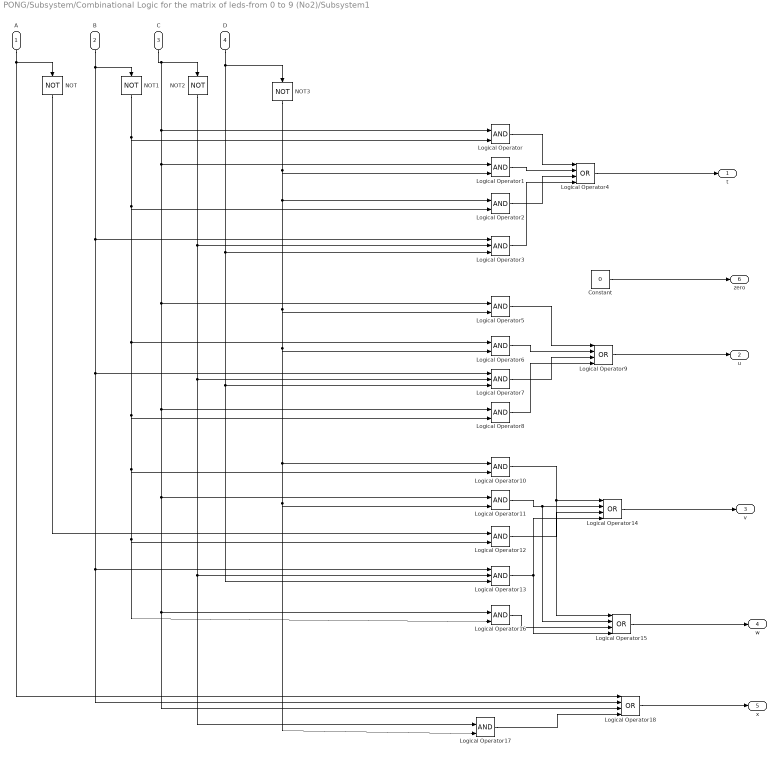
== system PONG/Subsystem/Combinational Logic for the matrix of leds-from 0 to 9 (No2)/Subsystem1 ==
  A : Inport
  B : Inport  Port=2
  C : Inport  Port=3
  D : Inport  Port=4
  Constant : Constant  Value=0  OutDataTypeStr=boolean
  Logical Operator{,1..2,5..6,8,10..12,16..17} (11 alike) : Logic  IconShape=distinctive  AllPortsSameDT=off  OutDataTypeStr=boolean
  Logical Operator13 : Logic  Inputs=3  IconShape=distinctive  AllPortsSameDT=off  OutDataTypeStr=boolean
  Logical Operator{4,9,14..15,18} (5 alike) : Logic  Operator=OR  Inputs=4  IconShape=distinctive  AllPortsSameDT=off  OutDataTypeStr=boolean
  Logical Operator3 : Logic  Inputs=3  IconShape=distinctive  AllPortsSameDT=off  OutDataTypeStr=boolean
  Logical Operator7 : Logic  Inputs=3  IconShape=distinctive  AllPortsSameDT=off  OutDataTypeStr=boolean
  NOT{,1..3} (4 alike) : Logic  Operator=NOT  IconShape=distinctive  AllPortsSameDT=off  OutDataTypeStr=boolean
  t : Outport
  u : Outport  Port=2
  v : Outport  Port=3
  w : Outport  Port=4
  x : Outport  Port=5
  zero : Outport  Port=6
  wires:
  A/1 -> Logical Operator18/1, NOT/1
  B/1 -> Logical Operator18/2, Logical Operator13/1, Logical Operator7/1, Logical Operator3/1, NOT1/1
  C/1 -> Logical Operator18/3, Logical Operator16/1, Logical Operator11/1, Logical Operator8/1, Logical Operator5/1, Logical Operator1/1, Logical Operator/1, NOT2/1
  D/1 -> Logical Operator13/3, Logical Operator7/3, Logical Operator3/3, NOT3/1
  NOT1/1 -> Logical Operator/2, Logical Operator2/2, Logical Operator16/2, Logical Operator12/2, Logical Operator10/2, Logical Operator8/2, Logical Operator6/1
  NOT3/1 -> Logical Operator1/2, Logical Operator2/1, Logical Operator17/2, Logical Operator11/2, Logical Operator10/1, Logical Operator6/2, Logical Operator5/2
  NOT2/1 -> Logical Operator17/1, Logical Operator13/2, Logical Operator7/2, Logical Operator3/2
  Logical Operator/1 -> Logical Operator4/1
  Logical Operator1/1 -> Logical Operator4/2
  Logical Operator2/1 -> Logical Operator4/3
  Logical Operator3/1 -> Logical Operator4/4
  Logical Operator4/1 -> t/1
  Logical Operator5/1 -> Logical Operator9/1
  Logical Operator6/1 -> Logical Operator9/2
  Logical Operator7/1 -> Logical Operator9/3
  Logical Operator8/1 -> Logical Operator9/4
  Logical Operator9/1 -> u/1
  Logical Operator10/1 -> Logical Operator15/1, Logical Operator14/1
  NOT/1 -> Logical Operator12/1
  Logical Operator12/1 -> Logical Operator14/3
  Logical Operator11/1 -> Logical Operator15/2, Logical Operator14/2
  Logical Operator13/1 -> Logical Operator15/4, Logical Operator14/4
  Logical Operator14/1 -> v/1
  Logical Operator15/1 -> w/1
  Logical Operator16/1 -> Logical Operator15/3
  Logical Operator17/1 -> Logical Operator18/4
  Logical Operator18/1 -> x/1
  Constant/1 -> zero/1

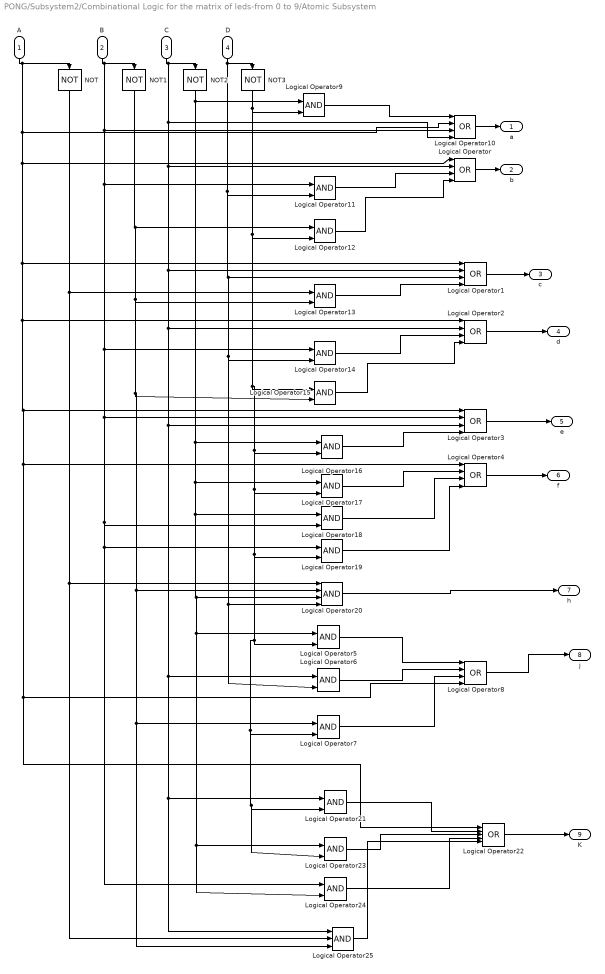
== system PONG/Subsystem2/Combinational Logic for the matrix of leds-from 0 to 9/Atomic Subsystem ==
  A : Inport
  B : Inport  Port=2
  C : Inport  Port=3
  D : Inport  Port=4
  Logical Operator{,1..4,8,10} (7 alike) : Logic  Operator=OR  Inputs=4  IconShape=distinctive  AllPortsSameDT=off  OutDataTypeStr=boolean
  Logical Operator{5..7,9,11..19,21,23..24} (16 alike) : Logic  IconShape=distinctive  AllPortsSameDT=off  OutDataTypeStr=boolean
  Logical Operator20 : Logic  Inputs=4  IconShape=distinctive  AllPortsSameDT=off  OutDataTypeStr=boolean
  Logical Operator22 : Logic  Operator=OR  Inputs=5  IconShape=distinctive  AllPortsSameDT=off  OutDataTypeStr=boolean
  Logical Operator25 : Logic  Inputs=3  IconShape=distinctive  AllPortsSameDT=off  OutDataTypeStr=boolean
  NOT{,1..3} (4 alike) : Logic  Operator=NOT  IconShape=distinctive  AllPortsSameDT=off  OutDataTypeStr=boolean
  a : Outport
  b : Outport  Port=2
  c : Outport  Port=3
  d : Outport  Port=4
  e : Outport  Port=5
  f : Outport  Port=6
  h : Outport  Port=7
  j : Outport  Port=8
  K : Outport  Port=9
  wires:
  Logical Operator8/1 -> j/1
  Logical Operator20/1 -> h/1
  Logical Operator12/1 -> Logical Operator/4
  A/1 -> Logical Operator8/4, Logical Operator22/1, Logical Operator4/1, Logical Operator3/1, Logical Operator2/1, Logical Operator1/1, Logical Operator/1, Logical Operator10/2, NOT/1
  Logical Operator3/1 -> e/1
  NOT1/1 -> Logical Operator25/3, Logical Operator7/1, Logical Operator20/2, Logical Operator15/2, Logical Operator13/2, Logical Operator12/1
  B/1 -> Logical Operator24/1, Logical Operator19/1, Logical Operator18/2, Logical Operator3/2, Logical Operator14/1, Logical Operator11/1, Logical Operator10/3, NOT1/1
  Logical Operator1/1 -> c/1
  Logical Operator4/1 -> f/1
  NOT2/1 -> Logical Operator24/2, Logical Operator23/1, Logical Operator5/1, Logical Operator20/3, Logical Operator18/1, Logical Operator17/1, Logical Operator16/1, Logical Operator9/1
  NOT3/1 -> Logical Operator19/2, Logical Operator23/2, Logical Operator21/2, Logical Operator7/2, Logical Operator5/2, Logical Operator17/2, Logical Operator16/2, Logical Operator15/1, Logical Operator12/2, Logical Operator9/2
  Logical Operator11/1 -> Logical Operator/3
  Logical Operator2/1 -> d/1
  D/1 -> Logical Operator6/2, Logical Operator20/4, Logical Operator14/2, Logical Operator1/3, Logical Operator11/2, NOT3/1
  Logical Operator9/1 -> Logical Operator10/1
  NOT/1 -> Logical Operator25/2, Logical Operator20/1, Logical Operator13/1
  Logical Operator13/1 -> Logical Operator1/4
  Logical Operator10/1 -> a/1
  Logical Operator/1 -> b/1
  Logical Operator14/1 -> Logical Operator2/3
  Logical Operator15/1 -> Logical Operator2/4
  Logical Operator16/1 -> Logical Operator3/4
  Logical Operator17/1 -> Logical Operator4/2
  Logical Operator18/1 -> Logical Operator4/3
  Logical Operator19/1 -> Logical Operator4/4
  Logical Operator5/1 -> Logical Operator8/1
  Logical Operator6/1 -> Logical Operator8/2
  Logical Operator7/1 -> Logical Operator8/3
  Logical Operator21/1 -> Logical Operator22/2
  Logical Operator23/1 -> Logical Operator22/3
  Logical Operator24/1 -> Logical Operator22/4
  Logical Operator22/1 -> K/1
  C/1 -> Logical Operator25/1, Logical Operator21/1, Logical Operator6/1, Logical Operator3/3, Logical Operator2/2, Logical Operator1/2, Logical Operator/2, Logical Operator10/4, NOT2/1
  Logical Operator25/1 -> Logical Operator22/5

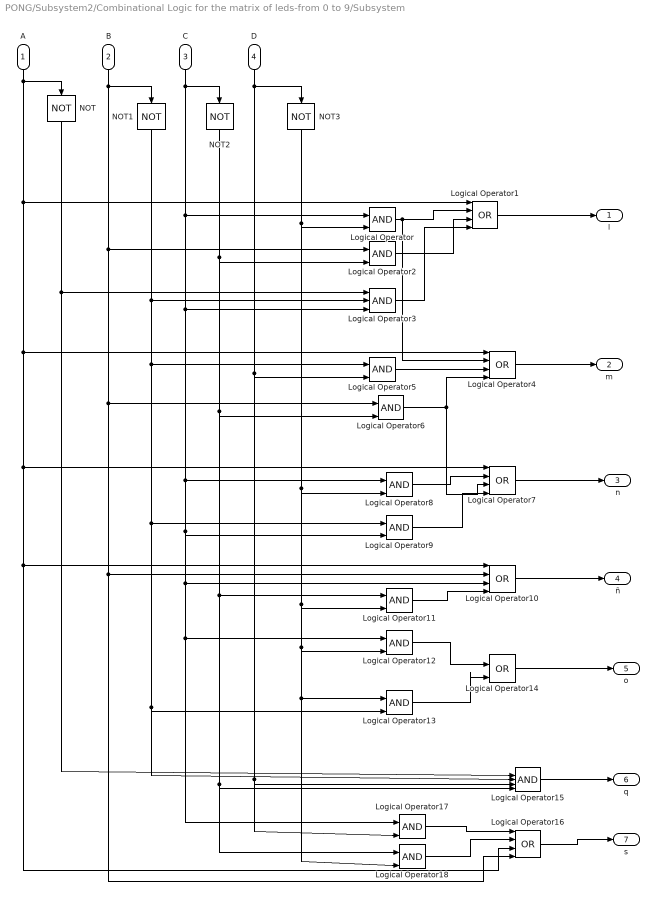
== system PONG/Subsystem2/Combinational Logic for the matrix of leds-from 0 to 9/Subsystem ==
  A : Inport
  B : Inport  Port=2
  C : Inport  Port=3
  D : Inport  Port=4
  Logical Operator{,2,5..6,8..9,11..13,17..18} (11 alike) : Logic  IconShape=distinctive  AllPortsSameDT=off  OutDataTypeStr=boolean
  Logical Operator{1,4,7,10,16} (5 alike) : Logic  Operator=OR  Inputs=4  IconShape=distinctive  AllPortsSameDT=off  OutDataTypeStr=boolean
  Logical Operator14 : Logic  Operator=OR  IconShape=distinctive  AllPortsSameDT=off  OutDataTypeStr=boolean
  Logical Operator15 : Logic  Inputs=4  IconShape=distinctive  AllPortsSameDT=off  OutDataTypeStr=boolean
  Logical Operator3 : Logic  Inputs=3  IconShape=distinctive  AllPortsSameDT=off  OutDataTypeStr=boolean
  NOT{,1..3} (4 alike) : Logic  Operator=NOT  IconShape=distinctive  AllPortsSameDT=off  OutDataTypeStr=boolean
  l : Outport
  m : Outport  Port=2
  n : Outport  Port=3
  ñ : Outport  Port=4
  o : Outport  Port=5
  q : Outport  Port=6
  s : Outport  Port=7
  wires:
  B/1 -> Logical Operator16/4, Logical Operator10/2, Logical Operator6/1, Logical Operator2/1, NOT1/1
  C/1 -> Logical Operator17/1, Logical Operator12/1, Logical Operator10/3, Logical Operator9/2, Logical Operator8/1, Logical Operator3/3, Logical Operator/1, NOT2/1
  D/1 -> Logical Operator17/2, Logical Operator15/3, Logical Operator5/2, NOT3/1
  NOT3/1 -> Logical Operator18/2, Logical Operator13/1, Logical Operator12/2, Logical Operator11/2, Logical Operator8/2, Logical Operator/2
  Logical Operator/1 -> Logical Operator4/2, Logical Operator1/2
  NOT2/1 -> Logical Operator18/1, Logical Operator15/4, Logical Operator11/1, Logical Operator6/2, Logical Operator2/2
  Logical Operator2/1 -> Logical Operator1/3
  NOT/1 -> Logical Operator15/1, Logical Operator3/1
  NOT1/1 -> Logical Operator15/2, Logical Operator13/2, Logical Operator9/1, Logical Operator5/1, Logical Operator3/2
  Logical Operator3/1 -> Logical Operator1/4
  A/1 -> Logical Operator16/3, Logical Operator10/1, Logical Operator7/1, Logical Operator4/1, Logical Operator1/1, NOT/1
  Logical Operator5/1 -> Logical Operator4/3
  Logical Operator6/1 -> Logical Operator7/3, Logical Operator4/4
  Logical Operator1/1 -> l/1
  Logical Operator4/1 -> m/1
  Logical Operator7/1 -> n/1
  Logical Operator8/1 -> Logical Operator7/2
  Logical Operator9/1 -> Logical Operator7/4
  Logical Operator11/1 -> Logical Operator10/4
  Logical Operator10/1 -> ñ/1
  Logical Operator12/1 -> Logical Operator14/1
  Logical Operator13/1 -> Logical Operator14/2
  Logical Operator14/1 -> o/1
  Logical Operator15/1 -> q/1
  Logical Operator17/1 -> Logical Operator16/1
  Logical Operator18/1 -> Logical Operator16/2
  Logical Operator16/1 -> s/1

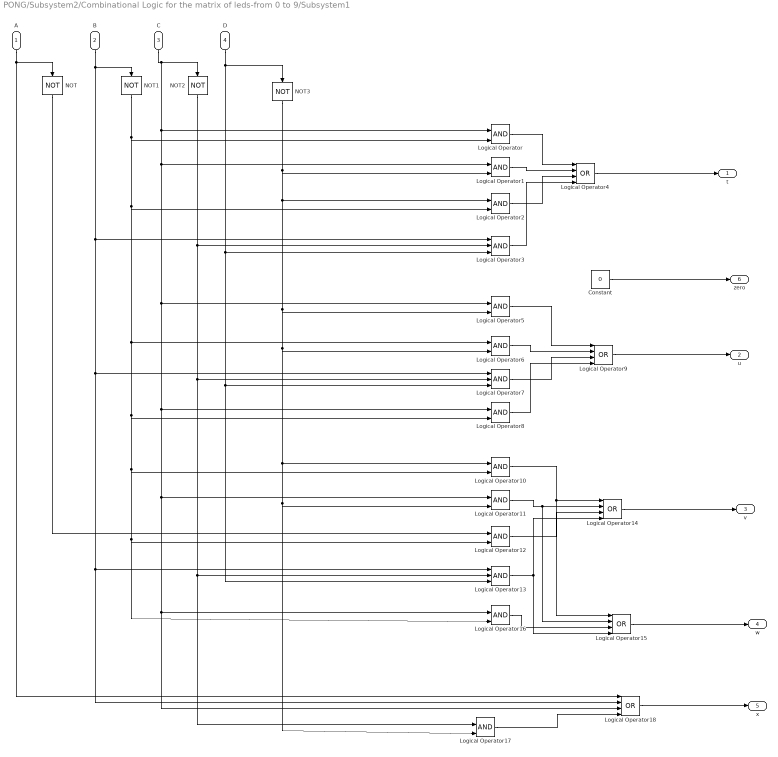
== system PONG/Subsystem2/Combinational Logic for the matrix of leds-from 0 to 9/Subsystem1 ==
  A : Inport
  B : Inport  Port=2
  C : Inport  Port=3
  D : Inport  Port=4
  Constant : Constant  Value=0  OutDataTypeStr=boolean
  Logical Operator{,1..2,5..6,8,10..12,16..17} (11 alike) : Logic  IconShape=distinctive  AllPortsSameDT=off  OutDataTypeStr=boolean
  Logical Operator13 : Logic  Inputs=3  IconShape=distinctive  AllPortsSameDT=off  OutDataTypeStr=boolean
  Logical Operator{4,9,14..15,18} (5 alike) : Logic  Operator=OR  Inputs=4  IconShape=distinctive  AllPortsSameDT=off  OutDataTypeStr=boolean
  Logical Operator3 : Logic  Inputs=3  IconShape=distinctive  AllPortsSameDT=off  OutDataTypeStr=boolean
  Logical Operator7 : Logic  Inputs=3  IconShape=distinctive  AllPortsSameDT=off  OutDataTypeStr=boolean
  NOT{,1..3} (4 alike) : Logic  Operator=NOT  IconShape=distinctive  AllPortsSameDT=off  OutDataTypeStr=boolean
  t : Outport
  u : Outport  Port=2
  v : Outport  Port=3
  w : Outport  Port=4
  x : Outport  Port=5
  zero : Outport  Port=6
  wires:
  A/1 -> Logical Operator18/1, NOT/1
  B/1 -> Logical Operator18/2, Logical Operator13/1, Logical Operator7/1, Logical Operator3/1, NOT1/1
  C/1 -> Logical Operator18/3, Logical Operator16/1, Logical Operator11/1, Logical Operator8/1, Logical Operator5/1, Logical Operator1/1, Logical Operator/1, NOT2/1
  D/1 -> Logical Operator13/3, Logical Operator7/3, Logical Operator3/3, NOT3/1
  NOT1/1 -> Logical Operator/2, Logical Operator2/2, Logical Operator16/2, Logical Operator12/2, Logical Operator10/2, Logical Operator8/2, Logical Operator6/1
  NOT3/1 -> Logical Operator1/2, Logical Operator2/1, Logical Operator17/2, Logical Operator11/2, Logical Operator10/1, Logical Operator6/2, Logical Operator5/2
  NOT2/1 -> Logical Operator17/1, Logical Operator13/2, Logical Operator7/2, Logical Operator3/2
  Logical Operator/1 -> Logical Operator4/1
  Logical Operator1/1 -> Logical Operator4/2
  Logical Operator2/1 -> Logical Operator4/3
  Logical Operator3/1 -> Logical Operator4/4
  Logical Operator4/1 -> t/1
  Logical Operator5/1 -> Logical Operator9/1
  Logical Operator6/1 -> Logical Operator9/2
  Logical Operator7/1 -> Logical Operator9/3
  Logical Operator8/1 -> Logical Operator9/4
  Logical Operator9/1 -> u/1
  Logical Operator10/1 -> Logical Operator15/1, Logical Operator14/1
  NOT/1 -> Logical Operator12/1
  Logical Operator12/1 -> Logical Operator14/3
  Logical Operator11/1 -> Logical Operator15/2, Logical Operator14/2
  Logical Operator13/1 -> Logical Operator15/4, Logical Operator14/4
  Logical Operator14/1 -> v/1
  Logical Operator15/1 -> w/1
  Logical Operator16/1 -> Logical Operator15/3
  Logical Operator17/1 -> Logical Operator18/4
  Logical Operator18/1 -> x/1
  Constant/1 -> zero/1
